simulink model "untitled"  (R2022b)
settings: Solver=ode4  StartTime=0.0  StopTime=7.5  FixedStep=0.0001  RelTol=1e-3
libraries: slrealtimeiplib x3, instrumentlib x3, slrealtimeutilitieslib x2
settings Model: PacingRate=1000  Creator=4qz  LastModifiedBy=4qz

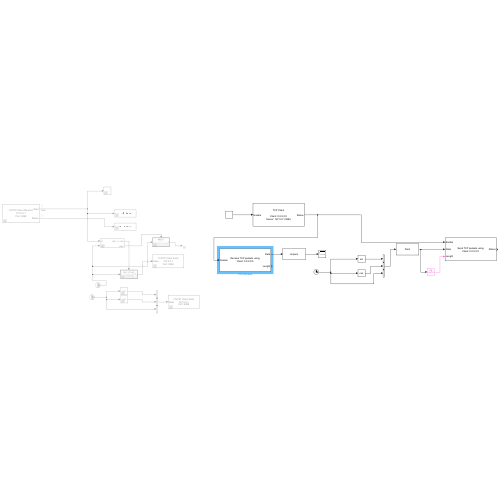
[thumbnail: Simulink's stored preview of the top-level diagram]
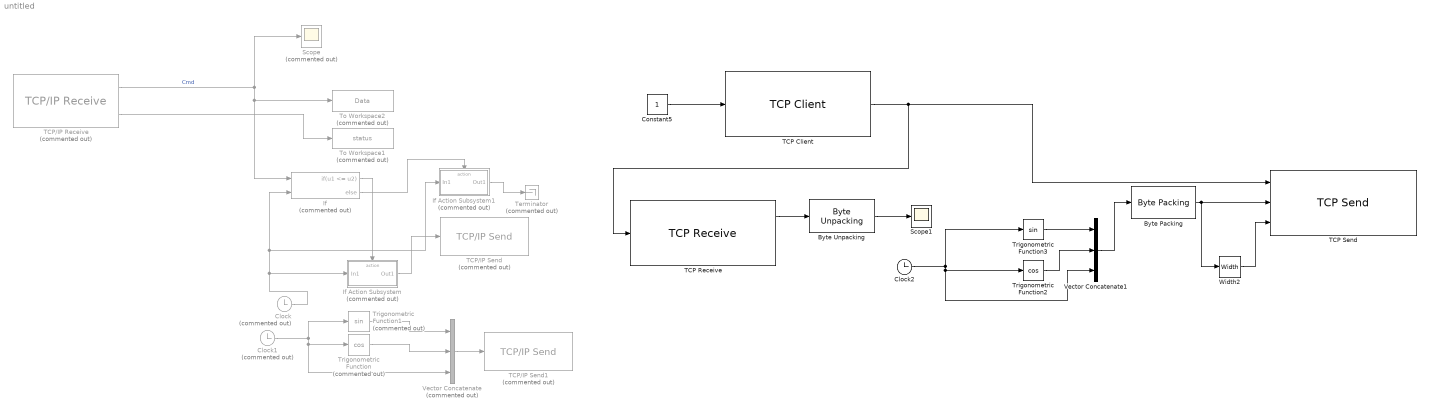
== system untitled ==
  Byte Packing : slrealtimeutilitieslib/Byte Packing  MaskPackedDataType=uint8  MaskUnpackedDataTypes={'double'}  MaskAlignment=1
  Byte Unpacking : slrealtimeutilitieslib/Byte Unpacking  MaskUnpackedDataTypes={'double'}  MaskUnpackedDataSizes={[1]}  MaskAlignment=1
  Clock : Clock  Commented=on
  Clock1 : Clock  Commented=on
  Clock2 : Clock
  Constant5 : Constant
  If : If  Commented=on  NumInputs=2  IfExpression=u1 <= u2
  If Action Subsystem : Subsystem  Commented=on  TreatAsAtomicUnit=on
  If Action Subsystem1 : Subsystem  Commented=on  TreatAsAtomicUnit=on
  Scope : Scope  Commented=on
  Scope1 : Scope
  TCP Client : slrealtimeiplib/TCP Client  Priority=-1  useHostTargetConn=off  remoteAddress=127.0.0.1  remotePort=9999
  TCP Receive : slrealtimeiplib/TCP Receive  socketAddPortVal=Client: 0.0.0.0:0  rcvWidth=8  sampleTime=0.0001
  TCP Send : slrealtimeiplib/TCP Send  socketAddPortVal=Client: 0.0.0.0:0  sampleTime=0.0001
  TCP/IP Receive : instrumentlib/TCP//IP Receive  Priority=1  Commented=on  Host=127.0.0.1  Port=9999  DataSize=[ 1, 1 ]  DataType=double  ASCIIFormatting=%f  Terminator=LF  CustomTerminator=10  ByteOrder=little-endian  EnableBlockingMode=off  Timeout=5  SampleTime=0.0001  SimulateUsing=Interpreted execution
  TCP/IP Send : instrumentlib/TCP//IP Send  Priority=2  Commented=on  Host=127.0.0.1  Port=9999  ByteOrder=little-endian  EnableBlockingMode=off  Timeout=0.1  TransferDelay=off  SimulateUsing=Interpreted execution
  TCP/IP Send1 : instrumentlib/TCP//IP Send  Priority=2  Commented=on  Host=127.0.0.1  Port=9999  ByteOrder=little-endian  EnableBlockingMode=off  Timeout=0.1  TransferDelay=off  SimulateUsing=Interpreted execution
  Terminator : Terminator  Commented=on
  To Workspace1 : ToWorkspace  Commented=on  VariableName=status  SampleTime=-1
      settings: Save2DSignal=2-D array (concatenate along first dimension)
  To Workspace2 : ToWorkspace  Commented=on  VariableName=Data  SampleTime=-1
      settings: Save2DSignal=2-D array (concatenate along first dimension)
  Trigonometric Function : Trigonometry  Commented=on  Operator=cos
  Trigonometric Function1 : Trigonometry  Commented=on
  Trigonometric Function2 : Trigonometry  Operator=cos
  Trigonometric Function3 : Trigonometry
  Vector Concatenate : Concatenate  Commented=on  NumInputs=3
  Vector Concatenate1 : Concatenate  NumInputs=3
  Width2 : Width
  wires:
  TCP/IP Receive/2 -> To Workspace1/1
  TCP/IP Receive/1 -> If/1, To Workspace2/1, Scope/1  "Cmd"
  Clock/1 -> If Action Subsystem/1(In1), If Action Subsystem1/1(In1), If/2
  If Action Subsystem/1(Out1) -> TCP/IP Send/1
  If/1 -> If Action Subsystem/Action
  If/2 -> If Action Subsystem1/Action
  If Action Subsystem1/1(Out1) -> Terminator/1
  Clock1/1 -> Trigonometric Function1/1, Vector Concatenate/3, Trigonometric Function/1
  Trigonometric Function/1 -> Vector Concatenate/2
  Vector Concatenate/1 -> TCP/IP Send1/1
  Trigonometric Function1/1 -> Vector Concatenate/1
  Constant5/1 -> TCP Client/1
  TCP Receive/1 -> Byte Unpacking/1
  Byte Unpacking/1 -> Scope1/1
  Width2/1 -> TCP Send/3
  Byte Packing/1 -> Width2/1, TCP Send/2
  TCP Client/1 -> TCP Receive/1, TCP Send/1
  Trigonometric Function3/1 -> Vector Concatenate1/1
  Clock2/1 -> Trigonometric Function3/1, Vector Concatenate1/3, Trigonometric Function2/1
  Vector Concatenate1/1 -> Byte Packing/1
  Trigonometric Function2/1 -> Vector Concatenate1/2

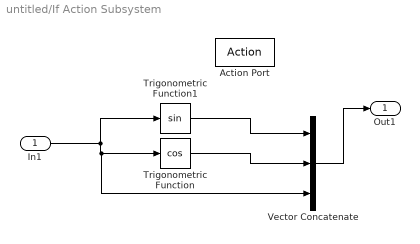
== system untitled/If Action Subsystem ==
  In1 : Inport
  Action Port : ActionPort  ActionPortLabel=if(u1 <= u2)
  Trigonometric Function : Trigonometry  Operator=cos
  Trigonometric Function1 : Trigonometry
  Vector Concatenate : Concatenate  NumInputs=3
  Out1 : Outport
  wires:
  In1/1 -> Trigonometric Function1/1, Vector Concatenate/3, Trigonometric Function/1
  Trigonometric Function/1 -> Vector Concatenate/2
  Trigonometric Function1/1 -> Vector Concatenate/1
  Vector Concatenate/1 -> Out1/1

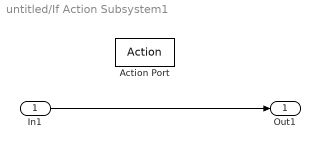
== system untitled/If Action Subsystem1 ==
  In1 : Inport
  Action Port : ActionPort  ActionPortLabel=else
  Out1 : Outport
  wires:
  In1/1 -> Out1/1
